simulink model "Problem5"  (R2020b)
settings: Solver=VariableStepAuto  StartTime=0.0  StopTime=10.0  RelTol=1e-3
settings Model: Creator=Shirish  LastModifiedBy=Shirish

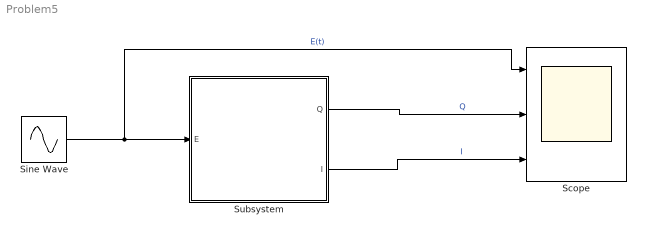
== system Problem5 ==
  Scope : Scope  NumInputPorts=3
  Sine Wave : Sin  Amplitude=5  Frequency=10  SampleTime=0
  Subsystem : Subsystem  mask{C=10^-5, R=10}
      mask prompts: C "Capacitance"; R "Resistance"
  wires:
  Sine Wave/1 -> Scope/1, Subsystem/1(E)  "E(t)"
  Subsystem/1(Q) -> Scope/2  "Q"
  Subsystem/2(I) -> Scope/3  "I"

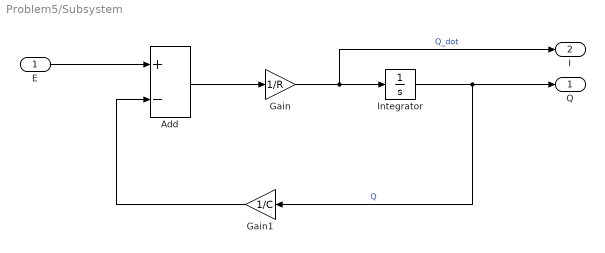
== system Problem5/Subsystem ==
  E : Inport
  Add : Sum  Inputs=+-
  Gain : Gain  Gain=1/R
  Gain1 : Gain  Gain=1/C
  Integrator : Integrator
  Q : Outport
  I : Outport  Port=2
  wires:
  Gain/1 -> I/1, Integrator/1  "Q_dot"
  E/1 -> Add/1
  Gain1/1 -> Add/2
  Integrator/1 -> Q/1, Gain1/1  "Q"
  Add/1 -> Gain/1
